simulink model "Channel"  (R2022a)
settings: Solver=VariableStepAuto  StartTime=0.0  StopTime=15  RelTol=1e-3
libraries: simulink x4, dspsigops x1, dspsrcs4 x1
(part 1 of 2)
settings Model: Creator=Sepiamw  LastModifiedBy=tina
settings DebuggingCC: UnconnectedInputMsg=warning  UnconnectedOutputMsg=warning  UnconnectedLineMsg=warning
settings RTWCC: DLArmComputeVersion=19.05

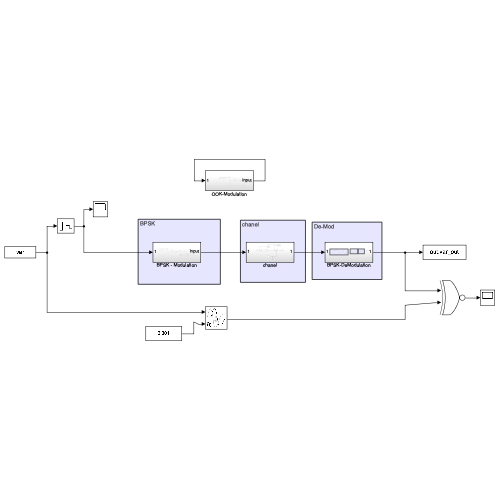
[thumbnail: Simulink's stored preview of the top-level diagram]
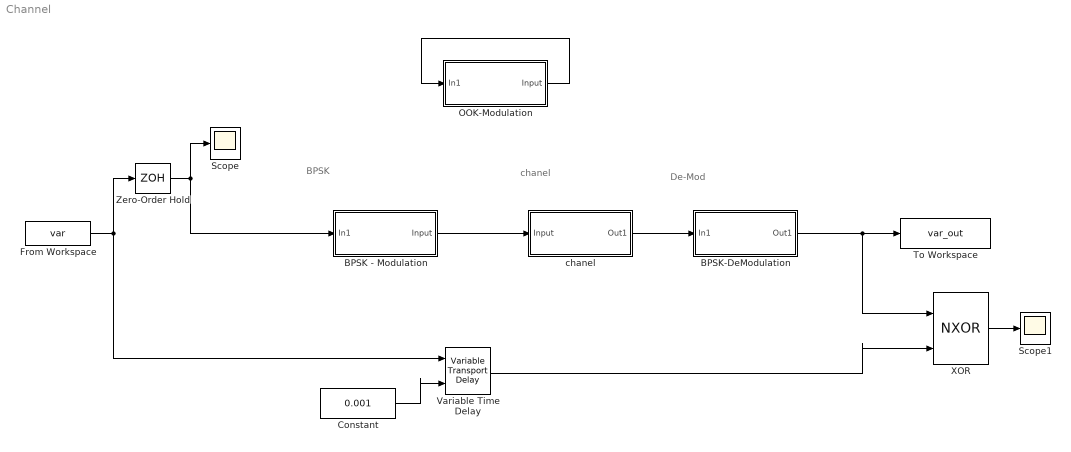
== system Channel ==
  note: De-Mod
  note: chanel
  note: BPSK
  BPSK - Modulation : Subsystem
  BPSK-DeModulation : Subsystem
  Constant : Constant  Value=0.001
  From Workspace : FromWorkspace  VariableName=var  OutDataTypeStr=double  SampleTime=1e-3
  OOK-Modulation : Subsystem
  Scope : Scope
  Scope1 : Scope
  To Workspace : ToWorkspace  VariableName=var_out  SampleTime=1e-5
      settings: Save2DSignal=2-D array (concatenate along first dimension)
  Variable Time Delay : VariableTransportDelay  MaximumDelay=10
  XOR : Logic  Operator=NXOR  IconShape=distinctive  AllPortsSameDT=off  OutDataTypeStr=boolean
  Zero-Order Hold : ZeroOrderHold  SampleTime=1e-3
  chanel : Subsystem
  wires:
  From Workspace/1 -> Variable Time Delay/1, Zero-Order Hold/1
  Zero-Order Hold/1 -> BPSK - Modulation/1(In1), Scope/1
  BPSK - Modulation/1(Input) -> chanel/1(Input)
  chanel/1(Out1) -> BPSK-DeModulation/1(In1)
  OOK-Modulation/1(Input) -> OOK-Modulation/1(In1)
  Constant/1 -> Variable Time Delay/2
  XOR/1 -> Scope1/1
  Variable Time Delay/1 -> XOR/2
  BPSK-DeModulation/1(Out1) -> To Workspace/1, XOR/1

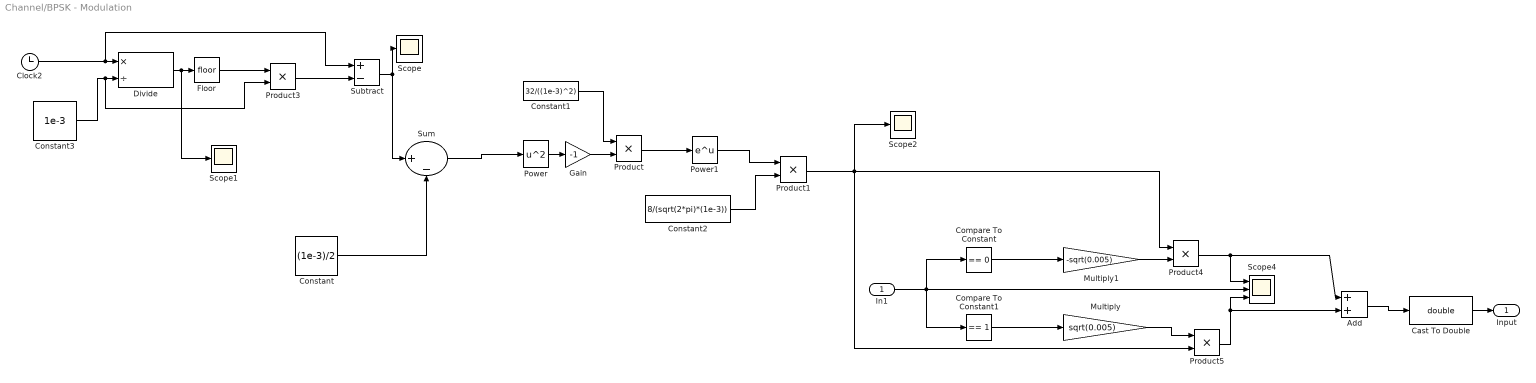
== system Channel/BPSK - Modulation ==
  In1 : Inport
  Add : Sum
  Cast To Double : DataTypeConversion  OutDataTypeStr=double  SaturateOnIntegerOverflow=off  RndMeth=Floor
  Clock2 : Clock
  Compare To Constant : simulink/Logic and Bit Operations/Compare To Constant  relop===  const=0  OutDataTypeStr=boolean
  Compare To Constant1 : simulink/Logic and Bit Operations/Compare To Constant  relop===  const=1  OutDataTypeStr=boolean
  Constant : Constant  Value=(1e-3)/2
  Constant1 : Constant  Value=32/((1e-3)^2)
  Constant2 : Constant  Value=8/(sqrt(2*pi)*(1e-3))
  Constant3 : Constant  Value=1e-3
  Divide : Product  Inputs=*/
  Floor : Rounding
  Gain : Gain  Gain=-1
  Multiply : Gain  Gain=sqrt(0.005)
  Multiply1 : Gain  Gain=-sqrt(0.005)
  Power : Math  Operator=square
  Power1 : Math
  Product{,1,3..5} (5 alike) : Product
  Scope : Scope
  Scope1 : Scope
  Scope2 : Scope
  Scope4 : Scope  NumInputPorts=3
  Subtract : Sum  Inputs=+-
  Sum : Sum  Inputs=|+-
  Input : Outport
  wires:
  Subtract/1 -> Scope/1, Sum/1
  Constant/1 -> Sum/2
  Sum/1 -> Power/1
  Power/1 -> Gain/1
  Constant1/1 -> Product/1
  Product/1 -> Power1/1
  Power1/1 -> Product1/1
  Constant2/1 -> Product1/2
  Product1/1 -> Product4/1, Product5/2, Scope2/1
  Gain/1 -> Product/2
  Clock2/1 -> Subtract/1, Divide/1
  Constant3/1 -> Product3/2, Divide/2
  Divide/1 -> Scope1/1, Floor/1
  Floor/1 -> Product3/1
  Product3/1 -> Subtract/2
  In1/1 -> Compare To Constant/1, Scope4/2, Compare To Constant1/1
  Compare To Constant/1 -> Multiply1/1
  Compare To Constant1/1 -> Multiply/1
  Multiply1/1 -> Product4/2
  Multiply/1 -> Product5/1
  Cast To Double/1 -> Input/1
  Product4/1 -> Add/1, Scope4/1
  Add/1 -> Cast To Double/1
  Product5/1 -> Scope4/3, Add/2

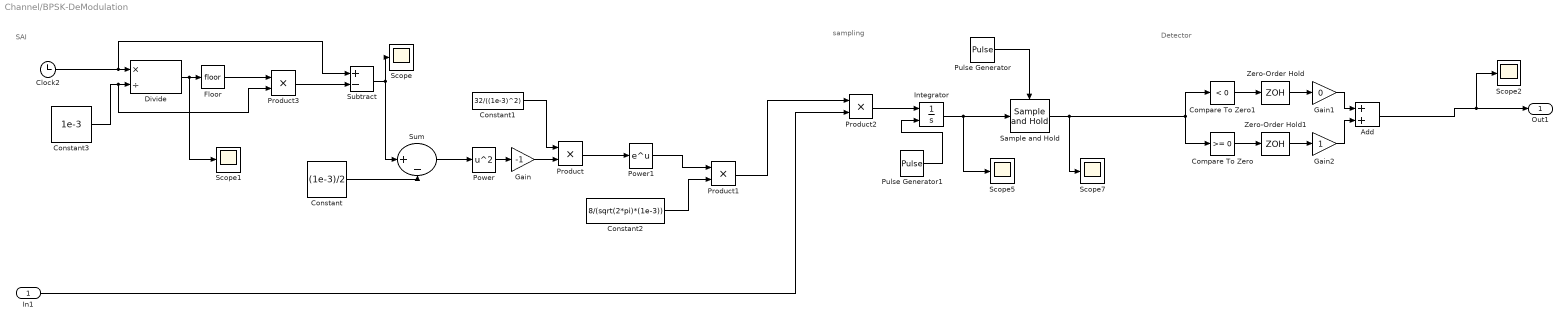
== system Channel/BPSK-DeModulation ==
  note: Detector
  note: sampling
  note: SAI
  In1 : Inport
  Add : Sum
  Clock2 : Clock
  Compare To Zero : simulink/Logic and Bit Operations/Compare To Zero  relop=>=  OutDataTypeStr=boolean
  Compare To Zero1 : simulink/Logic and Bit Operations/Compare To Zero  relop=<  OutDataTypeStr=boolean
  Constant : Constant  Value=(1e-3)/2
  Constant1 : Constant  Value=32/((1e-3)^2)
  Constant2 : Constant  Value=8/(sqrt(2*pi)*(1e-3))
  Constant3 : Constant  Value=1e-3
  Divide : Product  Inputs=*/
  Floor : Rounding
  Gain : Gain  Gain=-1
  Gain1 : Gain  Gain=0
  Gain2 : Gain
  Integrator : Integrator  ExternalReset=rising
  Power : Math  Operator=square
  Power1 : Math
  Product{,1..3} (4 alike) : Product
  Pulse Generator : DiscretePulseGenerator  PulseType=Time based  Period=1e-3  PulseWidth=50
  Pulse Generator1 : DiscretePulseGenerator  PulseType=Time based  Period=1e-3  PulseWidth=50
  Sample and Hold : dspsigops/Sample and Hold  trig=Falling edge  initCond=0  latchinput=off
  Scope{,1..2,5,7} (5 alike) : Scope
  Subtract : Sum  Inputs=+-
  Sum : Sum  Inputs=|+-
  Zero-Order Hold : ZeroOrderHold  SampleTime=1e-3
  Zero-Order Hold1 : ZeroOrderHold  SampleTime=1e-3
  Out1 : Outport
  wires:
  Product3/1 -> Subtract/2
  Divide/1 -> Scope1/1, Floor/1
  Constant3/1 -> Product3/2, Divide/2
  Power/1 -> Gain/1
  Product/1 -> Power1/1
  Subtract/1 -> Scope/1, Sum/1
  Power1/1 -> Product1/1
  Constant1/1 -> Product/1
  Gain/1 -> Product/2
  Clock2/1 -> Subtract/1, Divide/1
  Constant/1 -> Sum/2
  Constant2/1 -> Product1/2
  Floor/1 -> Product3/1
  Sum/1 -> Power/1
  Product1/1 -> Product2/1
  In1/1 -> Product2/2
  Integrator/1 -> Scope5/1, Sample and Hold/1
  Product2/1 -> Integrator/1
  Pulse Generator1/1 -> Integrator/2
  Pulse Generator/1 -> Sample and Hold/Trigger
  Gain1/1 -> Add/1
  Compare To Zero1/1 -> Zero-Order Hold/1
  Compare To Zero/1 -> Zero-Order Hold1/1
  Gain2/1 -> Add/2
  Sample and Hold/1 -> Compare To Zero/1, Compare To Zero1/1, Scope7/1
  Zero-Order Hold/1 -> Gain1/1
  Zero-Order Hold1/1 -> Gain2/1
  Add/1 -> Scope2/1, Out1/1

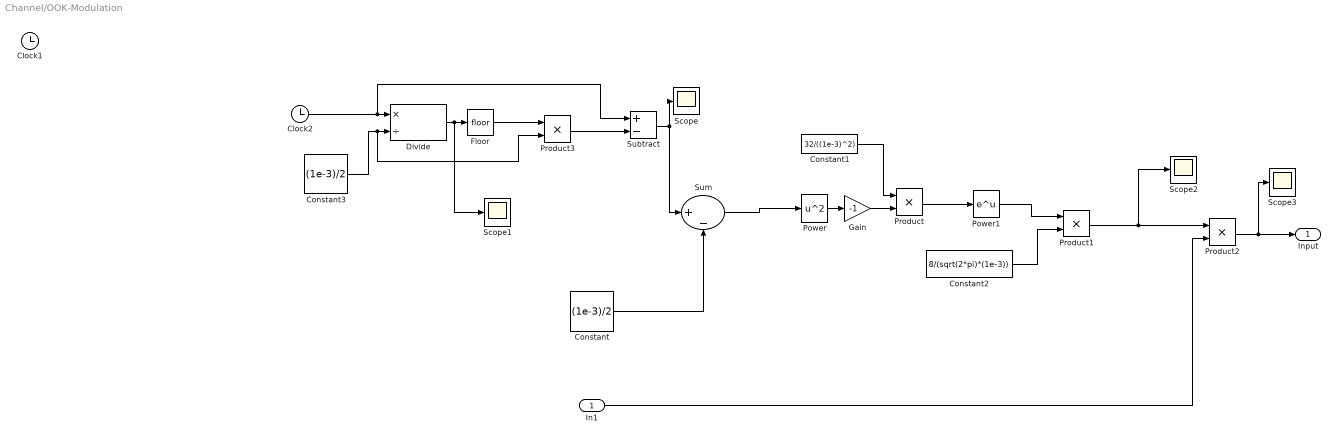
== system Channel/OOK-Modulation ==
  In1 : Inport
  Clock1 : Clock
  Clock2 : Clock
  Constant : Constant  Value=(1e-3)/2
  Constant1 : Constant  Value=32/((1e-3)^2)
  Constant2 : Constant  Value=8/(sqrt(2*pi)*(1e-3))
  Constant3 : Constant  Value=(1e-3)/2
  Divide : Product  Inputs=*/
  Floor : Rounding
  Gain : Gain  Gain=-1
  Power : Math  Operator=square
  Power1 : Math
  Product{,1..3} (4 alike) : Product
  Scope{,1..3} (4 alike) : Scope
  Subtract : Sum  Inputs=+-
  Sum : Sum  Inputs=|+-
  Input : Outport
  wires:
  Subtract/1 -> Scope/1, Sum/1
  Constant/1 -> Sum/2
  Sum/1 -> Power/1
  Power/1 -> Gain/1
  Constant1/1 -> Product/1
  Product/1 -> Power1/1
  Power1/1 -> Product1/1
  Constant2/1 -> Product1/2
  Product1/1 -> Scope2/1, Product2/1
  In1/1 -> Product2/2
  Product2/1 -> Scope3/1, Input/1
  Gain/1 -> Product/2
  Clock2/1 -> Subtract/1, Divide/1
  Constant3/1 -> Product3/2, Divide/2
  Divide/1 -> Scope1/1, Floor/1
  Floor/1 -> Product3/1
  Product3/1 -> Subtract/2

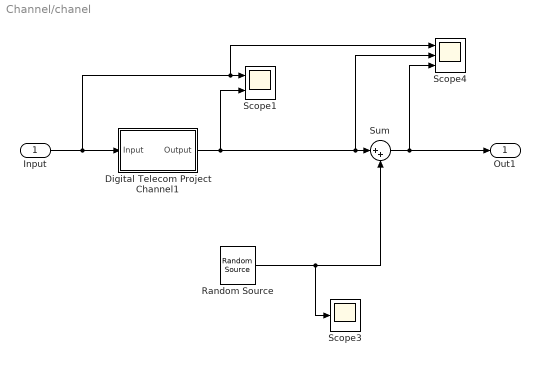
== system Channel/chanel ==
  Input : Inport
  Digital Telecom Project Channel1 : Subsystem  Tag=FilterWizardSubSystem
      settings: ErrorFcn=dspFilterRealizedInBasicElemsAlgLoopErrFcnCallback
  Random Source : dspsrcs4/Random Source  SrcType=Gaussian  NormMethod=Ziggurat  CltLength=12  MinVal=0  MaxVal=1  MeanVal=0  VarVal=5.4  RepMode=Not repeatable  rawSeed=1  IsInherit=off  SampMode=Discrete  SampTime=1e-5  SampFrame=1  DataType=Double  OutComplex=Real  OutputFrames=off
  Scope1 : Scope  NumInputPorts=2
  Scope3 : Scope
  Scope4 : Scope  NumInputPorts=3
  Sum : Sum  Inputs=|++
  Out1 : Outport
  wires:
  Digital Telecom Project Channel1/1(Output) -> Scope1/2, Scope4/2, Sum/1
  Sum/1 -> Scope4/3, Out1/1
  Random Source/1 -> Scope3/1, Sum/2
  Input/1 -> Scope4/1, Scope1/1, Digital Telecom Project Channel1/1(Input)
